simulink model "Turbine_JAM"  (R2024b)
settings: Solver=VariableStepAuto  StartTime=0.0  StopTime=10  RelTol=1e-3
libraries: slpidlib x1, simulink x1, aerolibpropulsion2 x1
settings Model: Creator=joleh  LastModifiedBy=joleh

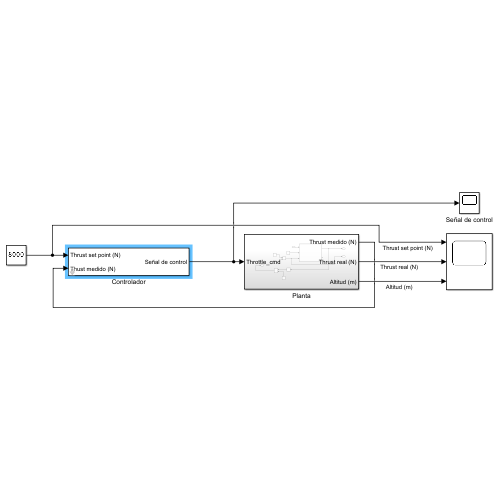
[thumbnail: Simulink's stored preview of the top-level diagram]
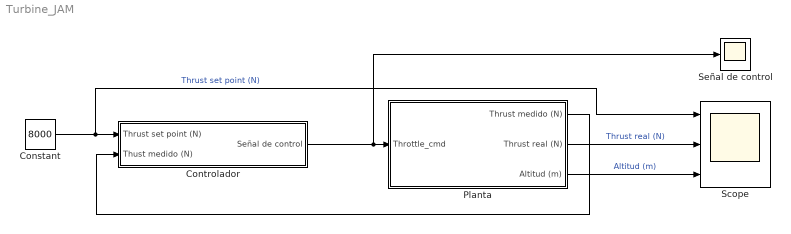
== system Turbine_JAM ==
  Constant : Constant  Value=8000
  Controlador : Subsystem  mask{kp_mask=0.001, ki_mask=0.005, kd_mask=0, tau=0.5}
      mask prompts: kp_mask "Kp"; ki_mask "Ki"; kd_mask "kd"; tau "Tau (válvula)"
  Planta : Subsystem
  Scope : Scope  NumInputPorts=3
  Señal de control : Scope
  wires:
  Constant/1 -> Controlador/1(Thrust set point (N)), Scope/1  "Thrust set point (N)"
  Controlador/1(Señal de control) -> Planta/1(Throttle_cmd), Señal de control/1
  Planta/1(Thrust medido (N)) -> Controlador/2(Thust medido (N))
  Planta/2(Thrust real (N)) -> Scope/2  "Thrust real (N)"
  Planta/3(Altitud (m)) -> Scope/3  "Altitud (m)"

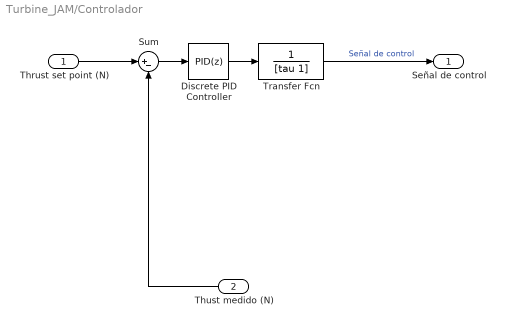
== system Turbine_JAM/Controlador ==
  Thrust set point (N) : Inport
  Thust medido (N) : Inport  Port=2
  Discrete PID Controller : slpidlib/PID Controller  Controller=PID  Form=Parallel  TimeDomain=Discrete-time  UseExternalTs=off  SampleTime=0.01  IntegratorMethod=Forward Euler  FilterMethod=Forward Euler  ControllerParametersSource=internal  P=kp_mask  I=ki_mask  UseKiTs=off  D=kd_mask  UseExternalDerivativeSource=off  N=100  UseFilter=on  TunerSelectOption=Transfer Function Based (PID Tuner App)  InitialConditionSource=internal  InitialConditionForIntegrator=0  InitialConditionForFilter=0  DifferentiatorICPrevScaledInput=0  ExternalReset=none  TrackingMode=off  Kt=1  LimitOutput=on  SatLimitsSource=internal  UpperSaturationLimit=1  LowerSaturationLimit=0  LinearizeAsGain=off  AntiWindupMode=clamping  Kb=1  LimitIntegrator=off  UpperIntegratorSaturationLimit=inf  LowerIntegratorSaturationLimit=-inf  POutMin=[]  POutMax=[]  IOutMin=[]  IOutMax=[]  DOutMin=[]  DOutMax=[]  NOutMin=[]  NOutMax=[]  SumOutMin=[]  SumOutMax=[]  SaturationOutMin=[]  SaturationOutMax=[]  PParamMin=[]  PParamMax=[]  IParamMin=[]  IParamMax=[]  DParamMin=[]  DParamMax=[]  NParamMin=[]  NParamMax=[]  KbParamMin=[]  KbParamMax=[]  KtParamMin=[]  KtParamMax=[]  KbOutMin=[]  KbOutMax=[]  KtOutMin=[]  KtOutMax=[]  IntegratorOutMin=[]  IntegratorOutMax=[]  FilterOutMin=[]  FilterOutMax=[]  SumI1OutMin=[]  SumI1OutMax=[]  SumI2OutMin=[]  SumI2OutMax=[]  SumI3OutMin=[]  SumI3OutMax=[]  SumI4OutMin=[]  SumI4OutMax=[]  SumDOutMin=[]  SumDOutMax=[]  DifferentiatorOutMin=[]  DifferentiatorOutMax=[]  FilterDiffOutCoefMin=[]  FilterDiffOutCoefMax=[]  ReciprocalOutMin=[]  ReciprocalOutMax=[]  SumDenOutMin=[]  SumDenOutMax=[]  SumNumOutMin=[]  SumNumOutMax=[]  DivideOutMin=[]  DivideOutMax=[]  UdiffTsProdOutMin=[]  UdiffTsProdOutMax=[]  NTsProdOutMin=[]  NTsProdOutMax=[]  UintegralTsProdOutMin=[]  UintegralTsProdOutMax=[]  UngainTsProdOutMin=[]  UngainTsProdOutMax=[]  ClampingZeroOutDataTypeStr=Inherit: Inherit via back propagation  ClampingZeroOutMin=[]  ClampingZeroOutMax=[]  FilterDenConstantOutDataTypeStr=Inherit: Inherit via back propagation  FilterDenConstantOutMin=[]  FilterDenConstantOutMax=[]  PCopyOutDataTypeStr=Inherit: Inherit via back propagation  PCopyOutMin=[]  PCopyOutMax=[]  NCopyOutDataTypeStr=Inherit: Inherit via back propagation  NCopyOutMin=[]  NCopyOutMax=[]  IntegratorContinuousStateAttributes=''  IntegratorStateMustResolveToSignalObject=off  IntegratorRTWStateStorageClass=Auto  FilterContinuousStateAttributes=''  FilterStateMustResolveToSignalObject=off  FilterRTWStateStorageClass=Auto  ParallelPVariant=InternalParameters  IdealPVariant=Disabled  IVariant=InternalParameters  DVariant=InternalParameters  IntegratorVariant=Discrete  SatVariant=Enabled  AWVariant=DiscClampingParallel  PCopyVariant=Disabled  TRVariant=Disabled  FdbkBlocksVariant=Forward  IdealPFdbkVariant=Disabled  SatFdbkVariant=Disabled  DerivativeFilterVariant=ForwardEulerFilter  NVariant=InternalParameters  NCopyVariant=Disabled  FilterICVariant=InternalICsFilter  IntegratorICVariant=InternalICs  ExternalResetVariant=Disabled  TRSumVariant=Passthrough  SumFdbkVariant=Disabled  SumVariant=Sum_PID  TsampFilterVariant=InternalTs  TsampNgainVariant=Passthrough  TsampIntegralVariant=Disabled_SignalSpec  ExternalSaturationOutDataTypeStr=Inherit: Same as second input  DerivativeSourceVariant=ErrorSignal  PreIntVariant=InternalPreInt
      settings: LibrarySourceBlock=simulink/Discrete/Discrete PID Controller
  Sum : Sum  Inputs=|+-
  Transfer Fcn : TransferFcn  Denominator=[tau 1]
  Señal de control : Outport
  wires:
  Sum/1 -> Discrete PID Controller/1
  Thrust set point (N)/1 -> Sum/1
  Thust medido (N)/1 -> Sum/2
  Transfer Fcn/1 -> Señal de control/1  "Señal de control"
  Discrete PID Controller/1 -> Transfer Fcn/1

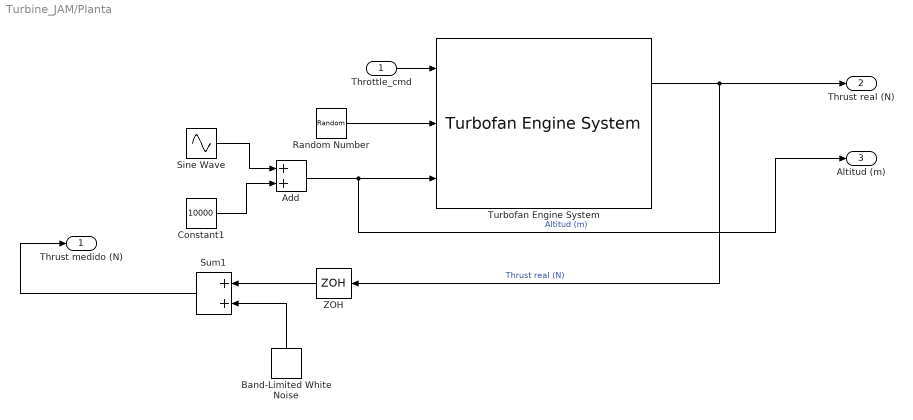
== system Turbine_JAM/Planta ==
  Throttle_cmd : Inport
  Add : Sum
  Band-Limited White Noise : simulink/Sources/Band-Limited White Noise  Cov=10  Ts=0.01  seed=[23341]
  Constant1 : Constant  Value=10000
  Random Number : RandomNumber  Mean=0.8  Variance=0.005  SampleTime=0.1
  Sine Wave : Sin  Amplitude=5  Frequency=5  SampleTime=0
  Sum1 : Sum
  Turbofan Engine System : aerolibpropulsion2/Turbofan Engine System  units=Metric (MKS)  ic_source=Internal  IC=0  Fmax=45000  tau=1  SFC=0.35  Nt=0.9
  ZOH : ZeroOrderHold  SampleTime=0.01
  Thrust medido (N) : Outport
  Thrust real (N) : Outport  Port=2
  Altitud (m) : Outport  Port=3
  wires:
  Random Number/1 -> Turbofan Engine System/2
  Constant1/1 -> Add/2
  Turbofan Engine System/1 -> Thrust real (N)/1, ZOH/1  "Thrust real (N)"
  Sine Wave/1 -> Add/1
  Band-Limited White Noise/1 -> Sum1/2
  ZOH/1 -> Sum1/1
  Add/1 -> Altitud (m)/1, Turbofan Engine System/3  "Altitud (m)"
  Sum1/1 -> Thrust medido (N)/1
  Throttle_cmd/1 -> Turbofan Engine System/1
